simulink model "FIR_Filter_4th_Order"  (R2020a)
settings: Solver=VariableStepAuto  StartTime=0.0  StopTime=10.0  RelTol=1e-3
settings Model: Creator=Viraj  LastModifiedBy=Viraj
settings DataIOCC: SaveOutput=off  SaveTime=off

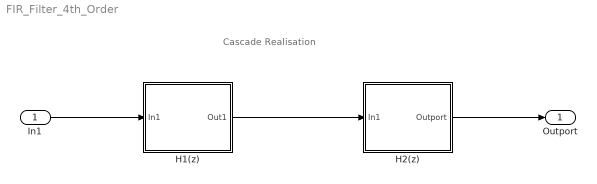
== system FIR_Filter_4th_Order ==
  note: Cascade Realisation
  In1 : Inport  OutDataTypeStr=double  PortDimensions=1  SampleTime=0
  H1(z) : Subsystem
  H2(z) : Subsystem
  Outport : Outport  OutDataTypeStr=double  PortDimensions=1  SampleTime=0
  wires:
  H1(z)/1(Out1) -> H2(z)/1(In1)
  H2(z)/1(Outport) -> Outport/1
  In1/1 -> H1(z)/1(In1)

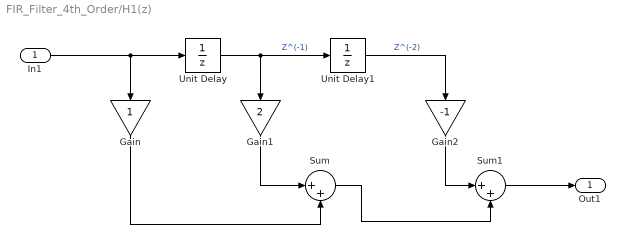
== system FIR_Filter_4th_Order/H1(z) ==
  In1 : Inport
  Gain : Gain
  Gain1 : Gain  Gain=2
  Gain2 : Gain  Gain=-1
  Sum : Sum  Inputs=|++
  Sum1 : Sum  Inputs=|++
  Unit Delay : UnitDelay  SampleTime=-1  HasFrameUpgradeWarning=on
  Unit Delay1 : UnitDelay  SampleTime=-1  HasFrameUpgradeWarning=on
  Out1 : Outport
  wires:
  Sum1/1 -> Out1/1
  Gain2/1 -> Sum1/1
  Sum/1 -> Sum1/2
  Unit Delay/1 -> Gain1/1, Unit Delay1/1  "Z^(-1)"
  In1/1 -> Gain/1, Unit Delay/1
  Gain/1 -> Sum/2
  Gain1/1 -> Sum/1
  Unit Delay1/1 -> Gain2/1  "Z^(-2)"

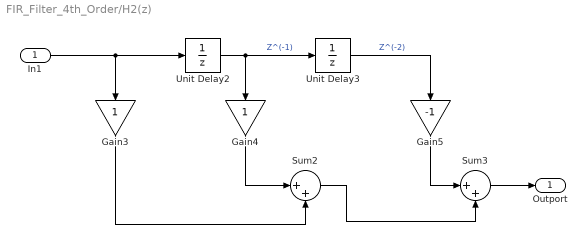
== system FIR_Filter_4th_Order/H2(z) ==
  In1 : Inport
  Gain3 : Gain
  Gain4 : Gain
  Gain5 : Gain  Gain=-1
  Sum2 : Sum  Inputs=|++
  Sum3 : Sum  Inputs=|++
  Unit Delay2 : UnitDelay  SampleTime=-1  HasFrameUpgradeWarning=on
  Unit Delay3 : UnitDelay  SampleTime=-1  HasFrameUpgradeWarning=on
  Outport : Outport
  wires:
  Sum3/1 -> Outport/1
  Gain4/1 -> Sum2/1
  Sum2/1 -> Sum3/2
  Gain3/1 -> Sum2/2
  Unit Delay2/1 -> Gain4/1, Unit Delay3/1  "Z^(-1)"
  Gain5/1 -> Sum3/1
  In1/1 -> Unit Delay2/1, Gain3/1
  Unit Delay3/1 -> Gain5/1  "Z^(-2)"
